simulink model "untitled"  (R2016b)
settings: Solver=VariableStepAuto  StartTime=0.0  StopTime=100.0  MaxStep=.01  RelTol=1e-3
settings Model: Creator=jesselayman  LastModifiedBy=jesselayman

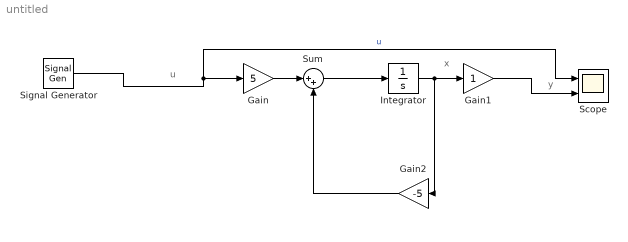
== system untitled ==
  note: y
  note: x
  note: u
  Gain : Gain  Gain=5
  Gain1 : Gain
  Gain2 : Gain  Gain=-5
  Integrator : Integrator
  Scope : Scope  NumInputPorts=2
  Signal Generator : SignalGenerator  Frequency=.1  Units=rad/sec
  Sum : Sum  Inputs=|++
  wires:
  Gain/1 -> Sum/1
  Sum/1 -> Integrator/1
  Integrator/1 -> Gain2/1, Gain1/1
  Gain2/1 -> Sum/2
  Gain1/1 -> Scope/2
  Signal Generator/1 -> Scope/1, Gain/1  "u"
